simulink model "miss4"  (Simulink 7.9)
settings: Solver=ode45  StartTime=0.0  StopTime=100  RelTol=1e-3
undefined symbols (not defined in the file or in its folder): L
libraries: simulink x2
settings Model: Creator=aziemba  LastModifiedBy=aziemba

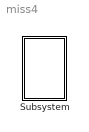
== system miss4 ==
  Subsystem : Subsystem  mask{t=0.1, t1=0.1, r=1, r1=3, m=2, k=5, l=2, g=9.81}

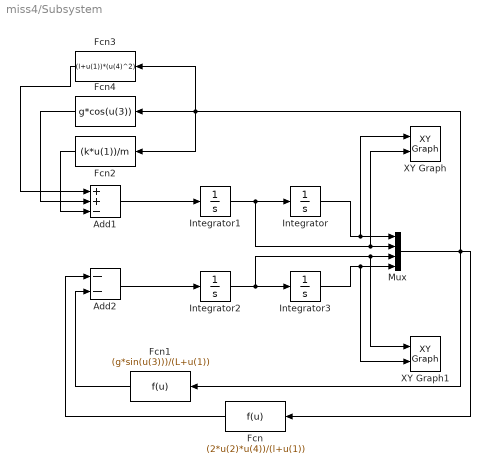
== system miss4/Subsystem ==
  Add1 : Sum  Inputs=++-
  Add2 : Sum  Inputs=--
  Fcn : Fcn  Expr=(2*u(2)*u(4))/(l+u(1))
  Fcn1 : Fcn  Expr=(g*sin(u(3)))/(L+u(1))
  Fcn2 : Fcn  Expr=(k*u(1))/m
  Fcn3 : Fcn  Expr=(l+u(1))*(u(4)^2)
  Fcn4 : Fcn  Expr=g*cos(u(3))
  Integrator : Integrator  InitialCondition=r
  Integrator1 : Integrator  InitialCondition=r1
  Integrator2 : Integrator  InitialCondition=t1
  Integrator3 : Integrator  InitialCondition=t
  Mux : Mux
  XY Graph : simulink/Sinks/XY Graph  xmin=-1  xmax=1  ymin=-1  ymax=1  st=-1
  XY Graph1 : simulink/Sinks/XY Graph  xmin=-1  xmax=1  ymin=-1  ymax=1  st=-1
  wires:
  Integrator2/1 -> Integrator3/1, Mux/3, XY Graph1/1
  Integrator1/1 -> Integrator/1, Mux/2, XY Graph/2
  Add1/1 -> Integrator1/1
  Add2/1 -> Integrator2/1
  Integrator/1 -> Mux/1, XY Graph/1
  Integrator3/1 -> Mux/4, XY Graph1/2
  Mux/1 -> Fcn/1, Fcn1/1, Fcn2/1, Fcn4/1, Fcn3/1
  Fcn/1 -> Add2/1
  Fcn1/1 -> Add2/2
  Fcn2/1 -> Add1/3
  Fcn4/1 -> Add1/2
  Fcn3/1 -> Add1/1
